simulink model "Laplace"  (R2015a)
settings: Solver=ode45  StartTime=0.0  StopTime=100  RelTol=1e-3
settings Model: Creator=ry0  LastModifiedBy=ry0

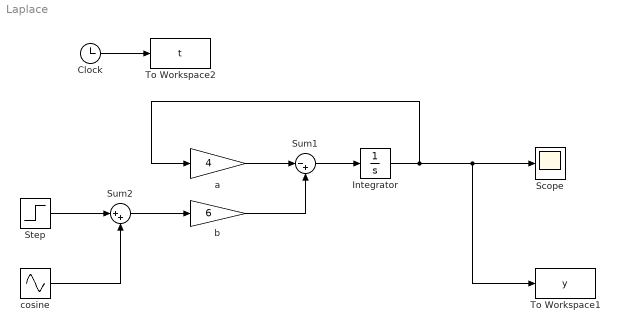
== system Laplace ==
  Clock : Clock
  Integrator : Integrator  InitialCondition=2
  Scope : Scope
  Step : Step  Time=0  SampleTime=0
  Sum1 : Sum  Inputs=|-+
  Sum2 : Sum  Inputs=|++
  To Workspace1 : ToWorkspace  VariableName=y  SampleTime=0.001
  To Workspace2 : ToWorkspace  VariableName=t  SampleTime=0.001
  a : Gain  Gain=4
  b : Gain  Gain=6
  cosine : Sin  Phase=pi/2  SampleTime=0
  wires:
  Sum1/1 -> Integrator/1
  Integrator/1 -> To Workspace1/1, Scope/1, a/1
  a/1 -> Sum1/1
  b/1 -> Sum1/2
  Sum2/1 -> b/1
  Step/1 -> Sum2/1
  cosine/1 -> Sum2/2
  Clock/1 -> To Workspace2/1
